simulink model "finalev"  (R2020b)
settings: Solver=VariableStepAuto  StartTime=0.0  StopTime=50  RelTol=1e-3  EnableMultiTasking=on
undefined symbols (not defined in the file): Ion, Lithium, sigbuilder_block
libraries: powerlib x27, simulink x6, electricdrivelib x2, re_lib x1
settings Model: Creator=lenovo  LastModifiedBy=rohan
settings DataIOCC: ReturnWorkspaceOutputs=off
settings OptimizationCC: LifeSpan=inf
settings DebuggingCC: SFUnexpectedBacktrackingDiag=warning  SFNoUnconditionalDefaultTransitionDiag=warning  ArithmeticOperatorsInVariantConditions=warning
settings SFSimCC: SimUseLocalCustomCode=off  CustomCodeUndefinedFunction=UseInterfaceOnly
settings RTWCC: RTWUseLocalCustomCode=off
settings CodeAppCC: StateflowObjectComments=on
settings GRTTargetCC: TargetLangStandard=C89/C90 (ANSI)
settings ConfigComp: CovMetricSettings=dw  CovSaveCumulativeToWorkspaceVar=on  CovSaveSingleToWorkspaceVar=on  CovExternalEMLEnable=off
settings SimscapeCC: SimscapeNormalizeSystem=off

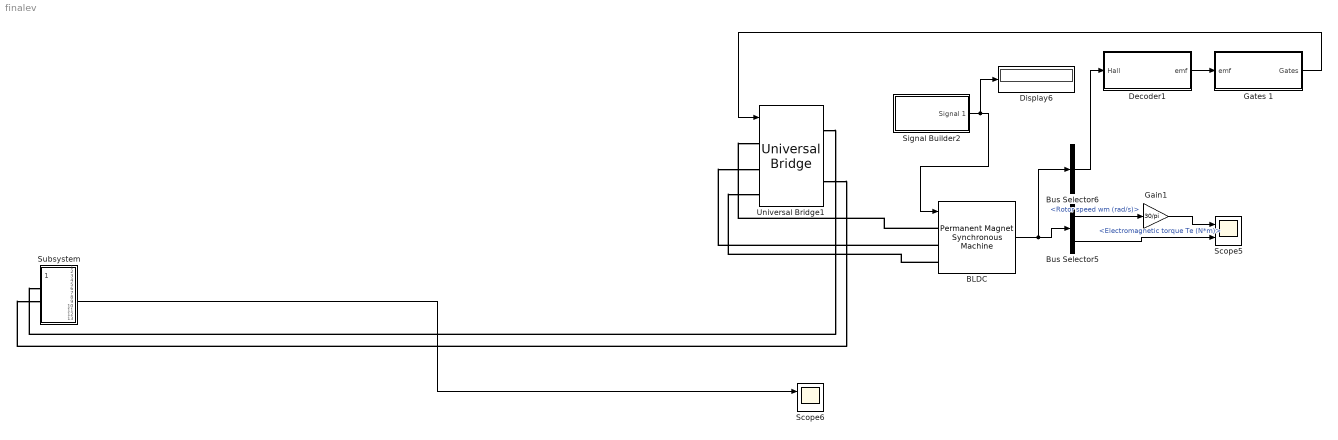
== system finalev ==
  BLDC : powerlib/Machines/Permanent Magnet Synchronous Machine  NbPhases=3  FluxDistribution=Trapezoidal  RotorType=Round  MechanicalLoad=Torque Tm  PresetModel=No  ShowDetailedParameters=on  MeasurementBus=off  Resistance=2.8750  Inductance=8.5e-3  dqInductances=[8.5e-3,8.5e-3]  La=0.000395  MachineConstant=Flux linkage established by magnets (V.s)  Flux=0.175  VoltageCst=146.6077  TorqueCst=1.4  Flat=120  Mechanical=[0.8e-3, 1e-3 4]  PolePairs=4  InitialConditions=[0,0, 0,0]  InitialConditions5ph=[0 0 0 0 0 0]  RefAngle=90 degrees behind phase A axis (modified Park)  IterativeDiscreteModel=Trapezoidal non iterative  TsBlock=-1  TsPowergui=0
  Bus Selector5 : BusSelector  OutputSignals=Rotor speed wm (rad/s),Electromagnetic torque Te (N*m)
  Bus Selector6 : BusSelector  OutputSignals=Hall effect signal h_a,Hall effect signal h_b,Hall effect signal h_c  OutputAsBus=on
  Decoder1 : Subsystem
  Display6 : Display
  Gain1 : Gain  Gain=30/pi
  Gates 1 : Subsystem
  Scope5 : Scope  NumInputPorts=2
  Scope6 : Scope  NumInputPorts=2
  Signal Builder2 : Subsystem  Tag=STV Subsys  LoadFcn=sigbuilder_block('load');  StartFcn=sigbuilder_block('start');  StopFcn=sigbuilder_block('stop');  ClipboardFcn=sigbuilder_block('clipboard');  mask(Sigbuilder block){tuvar=[0:10]}
      mask help: Simulink:masks:SigbuilderBlock_MD
      mask init:
      | if ~strcmp(get_param(bdroot(gcbh),'SimulationStatus'),'stopped') tuvar = sigbuilder_block('maskInit'); end
      settings: CopyFcn=sigbuilder_block('copy');  DeleteFcn=sigbuilder_block('delete');  ModelCloseFcn=sigbuilder_block('modelClose');  PreSaveFcn=sigbuilder_block('preSave');  PauseFcn=sigbuilder_block('pause');  ContinueFcn=sigbuilder_block('continue');  NameChangeFcn=sigbuilder_block('namechange');  OpenFcn=sigbuilder_block('open',[5.4 30 1141.2 522.6 ]);  CloseFcn=sigbuilder_block('close');
      mask Display: plot(0, 0, 100, 100,[2, 2, 32, 32, 2], [68, 8, 8, 68, 68],[32, 2], [38, 38], [32, 19, 2],[53, 60, 44], [32, 17, 17, 2],[16, 16, 31, 31]);txt = getActiveGroup(gcbh);text(2, 100, txt,'verticalAlignment', 'top');
  Subsystem : Subsystem
  Universal Bridge1 : powerlib/Power Electronics/Universal Bridge  Arms=3  SnubberResistance=5000  SnubberCapacitance=1e-6  Device=MOSFET / Diodes  Ron=1e-3  Lon=0  ForwardVoltages="[  0  0  ]"  ForwardVoltage=0  GTOparameters=[ 10e-6 , 20e-6 ]  IGBTparameters=[ 1e-6 , 2e-6 ]  Measurements=None  Measurements_2=None  converterType=Rectifier
  wires:
  Gain1/1 -> Scope5/1
  Bus Selector5/1 -> Gain1/1  "<Rotor speed wm (rad/s)>"
  Bus Selector6/1 -> Decoder1/1(Hall)
  Bus Selector5/2 -> Scope5/2  "<Electromagnetic torque Te (N*m)>"
  Gates 1/1("Gates ") -> Universal Bridge1/1
  Decoder1/1(emf) -> Gates 1/1(emf)
  BLDC/1 -> Bus Selector5/1, Bus Selector6/1
  Signal Builder2/1(Signal 1) -> Display6/1, BLDC/1
  Subsystem/9(Out9) -> Scope6/1
  connections:
  BLDC/LConn1 -- Universal Bridge1/LConn1
  BLDC/LConn2 -- Universal Bridge1/LConn2
  BLDC/LConn3 -- Universal Bridge1/LConn3
  Universal Bridge1/RConn1 -- Subsystem/LConn1
  Universal Bridge1/RConn2 -- Subsystem/LConn2

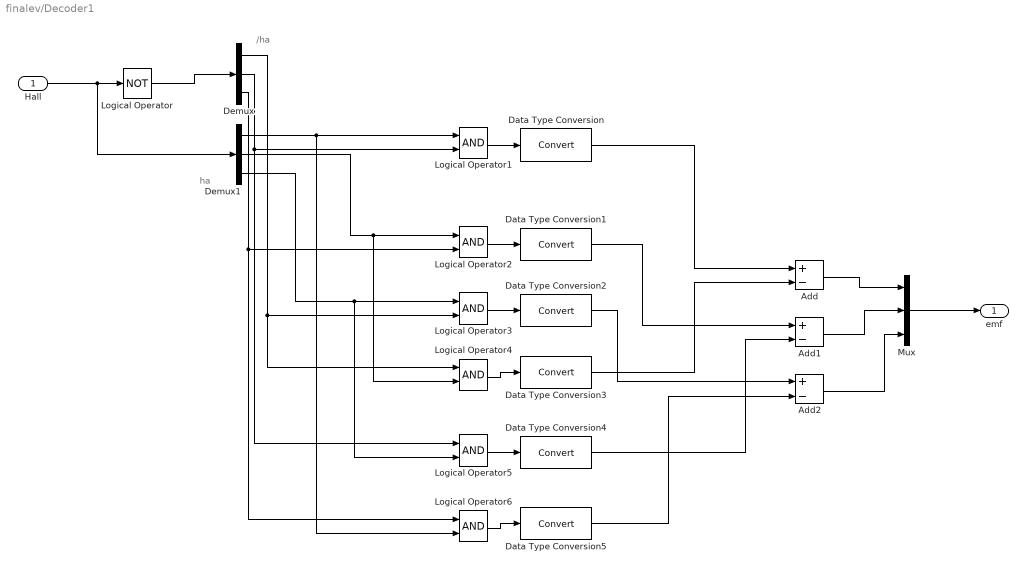
== system finalev/Decoder1 ==
  note: /ha
  note: ha
  Hall : Inport
  Add : Sum  Inputs=+-
  Add1 : Sum  Inputs=+-
  Add2 : Sum  Inputs=+-
  Data Type Conversion{,1..5} (6 alike) : DataTypeConversion
  Demux : Demux  Outputs=3
  Demux1 : Demux  Outputs=3
  Logical Operator : Logic  Operator=NOT  AllPortsSameDT=off  OutDataTypeStr=boolean
  Logical Operator{1..6} (6 alike) : Logic  AllPortsSameDT=off  OutDataTypeStr=boolean
  Mux : Mux  Inputs=3
  emf : Outport
  wires:
  Mux/1 -> emf/1
  Add2/1 -> Mux/3
  Add1/1 -> Mux/2
  Add/1 -> Mux/1
  Data Type Conversion5/1 -> Add2/2
  Data Type Conversion2/1 -> Add2/1
  Data Type Conversion4/1 -> Add1/2
  Data Type Conversion1/1 -> Add1/1
  Data Type Conversion3/1 -> Add/2
  Data Type Conversion/1 -> Add/1
  Logical Operator6/1 -> Data Type Conversion5/1
  Logical Operator5/1 -> Data Type Conversion4/1
  Logical Operator4/1 -> Data Type Conversion3/1
  Logical Operator3/1 -> Data Type Conversion2/1
  Logical Operator2/1 -> Data Type Conversion1/1
  Logical Operator1/1 -> Data Type Conversion/1
  Demux/3 -> Logical Operator6/1, Logical Operator2/2
  Demux/2 -> Logical Operator5/1, Logical Operator1/2
  Demux/1 -> Logical Operator4/1, Logical Operator3/2
  Demux1/3 -> Logical Operator3/1, Logical Operator5/2
  Demux1/2 -> Logical Operator2/1, Logical Operator4/2
  Demux1/1 -> Logical Operator1/1, Logical Operator6/2
  Logical Operator/1 -> Demux/1
  Hall/1 -> Logical Operator/1, Demux1/1

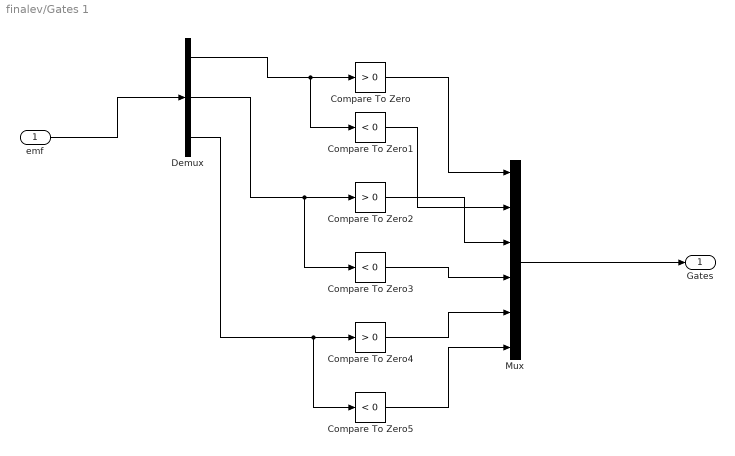
== system finalev/Gates 1 ==
  emf : Inport
  Compare To Zero : simulink/Logic and Bit Operations/Compare To Zero  relop=>  OutDataTypeStr=boolean
  Compare To Zero1 : simulink/Logic and Bit Operations/Compare To Zero  relop=<  OutDataTypeStr=boolean
  Compare To Zero2 : simulink/Logic and Bit Operations/Compare To Zero  relop=>  OutDataTypeStr=boolean
  Compare To Zero3 : simulink/Logic and Bit Operations/Compare To Zero  relop=<  OutDataTypeStr=boolean
  Compare To Zero4 : simulink/Logic and Bit Operations/Compare To Zero  relop=>  OutDataTypeStr=boolean
  Compare To Zero5 : simulink/Logic and Bit Operations/Compare To Zero  relop=<  OutDataTypeStr=boolean
  Demux : Demux  Outputs=3
  Mux : Mux  Inputs=6
  "Gates " : Outport
  wires:
  Mux/1 -> "Gates "/1
  Compare To Zero5/1 -> Mux/6
  Compare To Zero4/1 -> Mux/5
  Compare To Zero3/1 -> Mux/4
  Compare To Zero2/1 -> Mux/3
  Compare To Zero1/1 -> Mux/2
  Compare To Zero/1 -> Mux/1
  Demux/3 -> Compare To Zero4/1, Compare To Zero5/1
  Demux/2 -> Compare To Zero2/1, Compare To Zero3/1
  Demux/1 -> Compare To Zero/1, Compare To Zero1/1
  emf/1 -> Demux/1

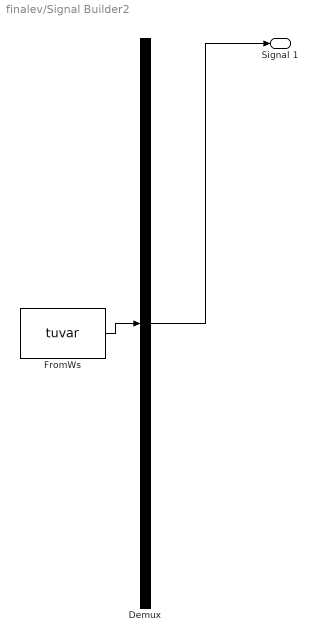
== system finalev/Signal Builder2 ==
  Demux : Demux  Tag=STV Demux  Outputs=1
      settings: DisplayOption=none
  FromWs : FromWorkspace  Tag=STV FromWs  VariableName=tuvar
      SigBuilderData=|
      | common.afterFinalStr = 'Extrapolate'
      | common.sampleTime = 0
      | dataSet.timeRange = [0 15]
      | dataSet.name = 'Group 1'
      | sbobj.Groups.Name = 'Group 1'
      | sbobj.Groups.Signals.Name = 'Signal 1'
      | sbobj.Groups.Signals.XData = [0 0.3 0.5 0.6 1 1.3 1.6 2 2.5 8 9 10 15]
      | sbobj.Groups.Signals.YData = [0.5 0.5 0.5 -0.3 -0.3 1 1 1 1.2 1 6.1 1.04 1.02]
      | sbobj.Groups.TimeRange = [0 15]
  Signal 1 : Outport  Tag=STV Outport
  wires:
  FromWs/1 -> Demux/1
  Demux/1 -> Signal 1/1

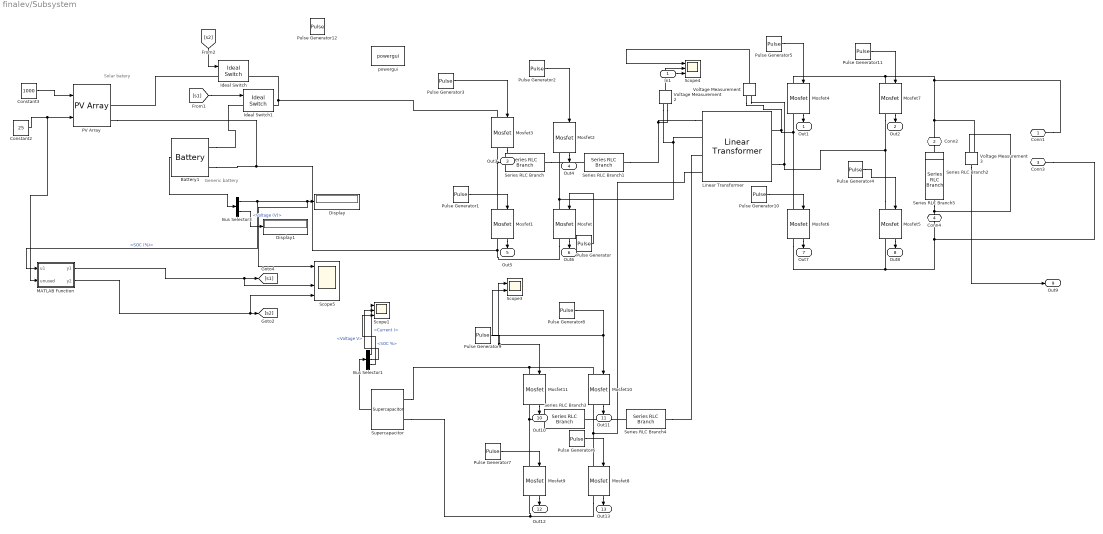
== system finalev/Subsystem ==
  note: Generic battery
  note: Solar batery
  In1 : Inport
  Battery1 : electricdrivelib/Extra Sources/Battery  BatType=Lithium-Ion  ShowTempParam=off  ThermalPreset=no  ShowAgeParam=off  NomV=48  NomQ=40  SOC=52  Batt_Tr=0.05  PresetModel=on  MaxQ=40  MinV=36  FullV=55.8714  Dis_rate=17.3913  R=0.012  Normal_OP=36.1739  expZone="[51.8585      1.96522]"  current=[6.5 13 32.5]  Units=Time  Tci=20  NomT=20  T2=-30  MaxQ2=4.8  FullV2=7.1  Normal_OP2=5.655  expZone2="[6.58           1]"  Rca=0.6  ti=2000  Dp=0  Neq0=0  Tsim=1e6  Ta1=25  Qeol=5.4*0.9  Reol=0.013333*1.2  Char_age=[2.3478, 3]  Dis_age=[2.3478, 10]  N1=1500  N2=10500  N3=1000  N4=1400  Ta2=45  N5=950
  Bus Selector1 : BusSelector  OutputSignals=Current I,Voltage V,SOC %
  Bus Selector3 : BusSelector  OutputSignals=SOC (%),Voltage (V)
  Constant2 : Constant  Value=25
  Constant3 : Constant  Value=1000
  Display : Display
  Display1 : Display
  Ideal Switch : powerlib/Power Electronics/Ideal Switch  Ron=0.001  Lon=0  IC=0  Rs=1e5  Cs=inf  Measurements=on
  Ideal Switch1 : powerlib/Power Electronics/Ideal Switch  Ron=0.001  Lon=0  IC=1  Rs=1e5  Cs=inf  Measurements=on
  Linear Transformer : powerlib/Elements/Linear Transformer  UNITS=pu  NominalPower=[ 500 100000]  winding1="[ 200  0.002  0.08 ]"  winding2="[ 50  0.002  0.08 ]"  ThreeWindings=on  winding3=[ 50 0.002 0.08 ]  RmLm=[ 10 10 ]  Measurements=None  DataType=off
  MATLAB Function : MATLAB Function  TreatAsAtomicUnit=on
  Mosfet{,1..11} (12 alike) : powerlib/Power Electronics/Mosfet  Ron=0.1  Lon=0  Rd=0.01  Vfd=0  IC=0  Rs=1e5  Cs=inf  Measurements=on
  PV Array : re_lib/Solar/PV Array  Npar=2  Nser=2  PlotType=array @ 25 deg.C & specified irradiances  S_vec="[ 1000  500  100 ]"  Temp_C_vec="[ 1000 500 100  ]"  ModuleName=User-defined  PlotWhenSelected=off  Pm=213.15  Ncell=60  Voc=36.3  Isc=7.84  Vm=29  Im=7.35  beta_Voc_pc=-0.36099  alpha_Isc_pc=0.102  beta_Voc=-0.13104  alpha_Isc=0.0079968  IL=7.8654  I0=2.9273e-10  nI=0.98119  Rsh=313.0553  Rs=0.39381  RobustModel=off  RobustCellTemperature=313.3991  BAL=on  Tc=1e-6  Tfilter=5e-5
  Pulse Generator{,3..6,9} (6 alike) : DiscretePulseGenerator  PulseType=Time based  Period=1/100e3  PulseWidth=50
  Pulse Generator{1..2,7..8,10..11} (6 alike) : DiscretePulseGenerator  PulseType=Time based  Period=1/100e3  PulseWidth=50  PhaseDelay=5e-6
  Pulse Generator12 : DiscretePulseGenerator  PulseType=Time based  Period=1/50  PulseWidth=60
  Scope1 : Scope  NumInputPorts=3
  Scope3 : Scope  NumInputPorts=2
  Scope4 : Scope  NumInputPorts=3
  Scope5 : Scope  NumInputPorts=4
  Series RLC Branch : powerlib/Elements/Series RLC Branch  LConnTagsString=__new0  RConnTagsString=__new0  BranchType=C  Resistance=1  Inductance=1e-3  SetiL0=off  InitialCurrent=0  Capacitance=0.1e-6  Setx0=off  InitialVoltage=0  Measurements=None
  Series RLC Branch1 : powerlib/Elements/Series RLC Branch  LConnTagsString=__new0  RConnTagsString=__new0  BranchType=L  Resistance=1  Inductance=28.44e-6  SetiL0=off  InitialCurrent=0  Capacitance=1e-6  Setx0=off  InitialVoltage=0  Measurements=None
  Series RLC Branch2 : powerlib/Elements/Series RLC Branch  LConnTagsString=__new0  RConnTagsString=__new0  BranchType=C  Resistance=1  Inductance=1e-3  SetiL0=off  InitialCurrent=0  Capacitance=0.5e-6  Setx0=off  InitialVoltage=0  Measurements=None
  Series RLC Branch3 : powerlib/Elements/Series RLC Branch  LConnTagsString=__new0  RConnTagsString=__new0  BranchType=C  Resistance=1  Inductance=1e-3  SetiL0=off  InitialCurrent=0  Capacitance=0.22e-6  Setx0=off  InitialVoltage=0  Measurements=None
  Series RLC Branch4 : powerlib/Elements/Series RLC Branch  LConnTagsString=__new0  RConnTagsString=__new0  BranchType=L  Resistance=1  Inductance=15e-6  SetiL0=off  InitialCurrent=0  Capacitance=1e-6  Setx0=off  InitialVoltage=0  Measurements=None
  Series RLC Branch5 : powerlib/Elements/Series RLC Branch  LConnTagsString=__new0  RConnTagsString=__new0  BranchType=C  Resistance=1  Inductance=1e-3  SetiL0=off  InitialCurrent=0  Capacitance=0.5e-6  Setx0=off  InitialVoltage=0  Measurements=None
  Supercapacitor : electricdrivelib/Extra Sources/Supercapacitor  C=40  Rdc=20e-3  Voltage=35  Ns=182  Np=18  Vinit=35  Temp=25  PresetModel=off  EstParam=off  Nc=1  r=1e-9  epsilon=6.0208e-10  Ich=10  Vstern="[0.161  2.7  7.8]"  Self_dis=on  Ioc=10  Vself="[48  47.8  47.06  44.65]"  demandeplot=off  I="[10  20 100  500]"  Units=sec  Vmax=0  If=0  deltaV=0  alpha=0  sec=0
      settings: SourceProductBaseCode=PS
  Voltage Measurement : powerlib/Measurements/Voltage Measurement  PhasorSimulation=off  OutputType=Complex  PSBequivalent=0
  Voltage Measurement2 : powerlib/Measurements/Voltage Measurement  PhasorSimulation=off  OutputType=Complex  PSBequivalent=0
  Voltage Measurement3 : powerlib/Measurements/Voltage Measurement  PhasorSimulation=off  OutputType=Complex  PSBequivalent=0
  powergui : powerlib/powergui  Priority=1  SimulationMode=Discrete  SampleTime=50e-7  frequency=60  Iterations=50  frequencyindice=0  Pbase=100e6  ErrMax=1e-4  UnitsV=kV  UnitsW=MW  buscounter=0  FunctionMessages=off  echomessages=off  EnableUseOfTLC=off  CurrentSourceSwitches=off  DisableSnubberDevices=off  DisableRonSwitches=off  DisableVfSwitches=off  DisplayEquations=off  AutomaticDiscreteSolvers=off  SolverType=Tustin/Backward Euler (TBE)  Interpol=off  ExternalGateDelay=off  methode=off  Ts=10  x0status=blocks  SPID=off  SwTol=0  HookPort=off  NonlinearTolerance=1e-4  nMaxIteration=100  ContinueOnMaxIteration=off  RestoreLinks=warning  ResistiveCurrentMeasurement=off  Frange=[0:2:500]  Ylog=off  Xlog=on  ShowGrid=off  save=off  variable=ZData  structure=0  ZoomFFT=off  StartTime=0.0  cycles=1  DisplayStyle=1  fundamental=60  FreqAxis=off  MaxFrequency=1000  frequencyindicesteady=1  RmsSteady=1  display=off
  Conn1 : PMIOPort  Side=Left
  Conn2 : PMIOPort  Port=2  Side=Right
  Conn3 : PMIOPort  Port=3  Side=Left
  Conn4 : PMIOPort  Port=4  Side=Left
  Out1 : Outport
  Out2 : Outport  Port=2
  Out3 : Outport  Port=3
  Out4 : Outport  Port=4
  Out5 : Outport  Port=5
  Out6 : Outport  Port=6
  Out7 : Outport  Port=7
  Out8 : Outport  Port=8
  Out9 : Outport  Port=9
  Out10 : Outport  Port=10
  Out11 : Outport  Port=11
  Out12 : Outport  Port=12
  Out13 : Outport  Port=13
  wires:
  Mosfet/1 -> Out6/1
  Mosfet9/1 -> Out12/1
  Mosfet7/1 -> Out2/1
  Mosfet2/1 -> Out4/1
  Mosfet8/1 -> Out13/1
  Mosfet11/1 -> Out10/1
  Mosfet1/1 -> Out5/1
  Mosfet10/1 -> Out11/1
  Mosfet6/1 -> Out7/1
  Mosfet5/1 -> Out8/1
  Mosfet4/1 -> Out1/1
  In1/1 -> Scope4/3
  Mosfet3/1 -> Out3/1
  Pulse Generator2/1 -> Mosfet2/1
  Voltage Measurement2/1 -> Scope4/2
  Pulse Generator6/1 -> Mosfet8/1
  Bus Selector1/1 -> Scope1/1  "<Current I>"
  Pulse Generator11/1 -> Mosfet7/1
  Pulse Generator10/1 -> Mosfet6/1
  Bus Selector1/3 -> Scope1/3  "<SOC %>"
  Pulse Generator9/1 -> Mosfet11/1, Scope3/1
  Pulse Generator1/1 -> Mosfet1/1
  Pulse Generator4/1 -> Mosfet5/1
  Pulse Generator/1 -> Mosfet/1
  Pulse Generator8/1 -> Scope3/2, Mosfet10/1
  Voltage Measurement/1 -> Scope4/1
  Supercapacitor/1 -> Bus Selector1/1
  Bus Selector1/2 -> Scope1/2  "<Voltage V>"
  Pulse Generator3/1 -> Mosfet3/1
  Pulse Generator7/1 -> Mosfet9/1
  Pulse Generator5/1 -> Mosfet4/1
  Voltage Measurement3/1 -> Out9/1
  Battery1/1 -> Bus Selector3/1
  Bus Selector3/1 -> Scope5/1, Display/1, MATLAB Function/1(u1)  "<SOC (%)>"
  Bus Selector3/2 -> Display1/1  "<Voltage (V)>"
  [s2] -> Ideal Switch/1
  [s1] -> Ideal Switch1/1
  MATLAB Function/1(y1) -> Scope5/3, [s1]
  MATLAB Function/2(y2) -> Scope5/4, [s2]
  ? -> ?
  Constant2/1 -> MATLAB Function/2(unused), PV Array/2
  Constant3/1 -> PV Array/1
  connections:
  Series RLC Branch5/LConn1 -- Conn2/RConn1
  Series RLC Branch5/RConn1 -- Conn4/RConn1
  Mosfet5/RConn1 -- Conn3/RConn1 -- Voltage Measurement3/LConn2 -- Series RLC Branch2/RConn1 -- Mosfet6/RConn1
  Linear Transformer/RConn4 -- Series RLC Branch1/RConn1 -- Voltage Measurement2/LConn2
  Mosfet2/RConn1 -- Mosfet/LConn1 -- Linear Transformer/RConn3 -- Voltage Measurement2/LConn1
  Mosfet10/LConn1 -- Supercapacitor/LConn1 -- Mosfet11/LConn1
  Mosfet5/LConn1 -- Mosfet7/RConn1 -- Linear Transformer/LConn1 -- Voltage Measurement/LConn2
  Mosfet8/RConn1 -- Supercapacitor/LConn2 -- Mosfet9/RConn1
  Battery1/LConn2 -- PV Array/RConn2 -- Mosfet/RConn1 -- Mosfet1/RConn1
  Mosfet8/LConn1 -- Mosfet10/RConn1 -- Linear Transformer/RConn1
  Mosfet4/RConn1 -- Mosfet6/LConn1 -- Voltage Measurement/LConn1 -- Linear Transformer/LConn2
  Mosfet3/RConn1 -- Mosfet1/LConn1 -- Series RLC Branch/LConn1
  Mosfet11/RConn1 -- Mosfet9/LConn1 -- Series RLC Branch3/LConn1
  Series RLC Branch/RConn1 -- Series RLC Branch1/LConn1
  Series RLC Branch4/LConn1 -- Series RLC Branch3/RConn1
  Mosfet7/LConn1 -- Conn1/RConn1 -- Voltage Measurement3/LConn1 -- Series RLC Branch2/LConn1 -- Mosfet4/LConn1
  Series RLC Branch4/RConn1 -- Linear Transformer/RConn2
  Ideal Switch/RConn1 -- Mosfet3/LConn1 -- Ideal Switch1/RConn1
  Ideal Switch/LConn1 -- PV Array/RConn1
  Battery1/LConn1 -- Ideal Switch1/LConn1

== matlab function finalev/Subsystem/MATLAB Function ==
  data: u1 input; y1 output; unused input; y2 output
function [y1,y2] = fcn(u1,~)
if u1>50.367
    y1=1;
    y2=0;
else
    y1=0;
    y2=1;
end
